simulink model "ServoModel2"  (Simulink 7.3)
settings: Solver=ode45  StartTime=0.0  StopTime=4  RelTol=1e-3
settings Model: Creator=Sainquake Notebook  LastModifiedBy=Sainquake Notebook

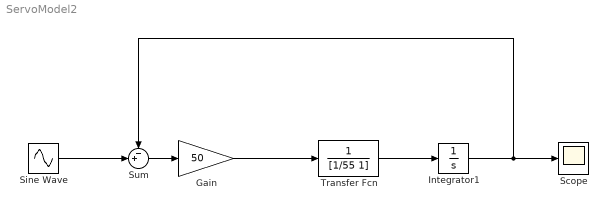
== system ServoModel2 ==
  Gain : Gain  Gain=50  ParameterDataType=fixdt(1, 16)  ParameterScaling=2^0  OutDataType=fixdt(1, 16)  OutScaling=2^0
  Integrator1 : Integrator
  Scope : Scope
  Sine Wave : Sin  Amplitude=1  Bias=0  Frequency=120  Phase=0  Samples=10  SampleTime=0  Offset=0
  Sum : Sum  Inputs=-+|  OutDataType=fixdt(1, 16)  OutScaling=2^0
  Transfer Fcn : TransferFcn  Denominator=[1/55 1]
  wires:
  Gain/1 -> Transfer Fcn/1
  Sum/1 -> Gain/1
  Sine Wave/1 -> Sum/2
  Integrator1/1 -> Sum/1, Scope/1
  Transfer Fcn/1 -> Integrator1/1
